simulink model "step2"  (R2018a)
settings: Solver=ode45  StartTime=0.0  StopTime=4  RelTol=1e-3
values from neighbouring files (symbols this model uses):
  Beta = 0    [step2.m]
  Friction = 22600    [step2.m]
  Inertia = 250000    [step2.m]
  Lambdam = 14.3522    [step2.m]
  Ld = 0.0035218    [step2.m]
  Lq = 0.0035218    [step2.m]
  Pole = 118    [step2.m]
  R = 58    [step2.m]
  Ro = 1.225    [step2.m]
  Rs = 0.05    [step2.m]
  Vw = 11.8    [step2.m]
libraries: powerlib x17, peTransforms x2
settings Model: Creator=Xinyi Zhang  LastModifiedBy=zxyxi

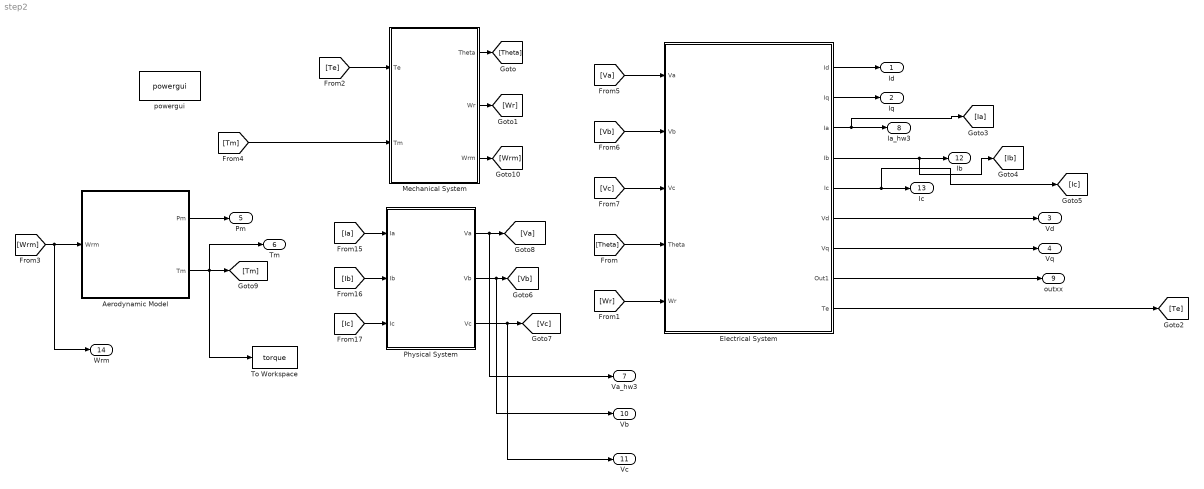
== system step2 ==
  "Aerodynamic Model " : Subsystem
  "Electrical System " : Subsystem
  "Mechanical System " : Subsystem
  "Physical System " : Subsystem
  To Workspace : ToWorkspace  VariableName=torque  SaveFormat=Timeseries  SampleTime=-1
  powergui : powerlib/powergui  Priority=1  SimulationMode=Discrete  SampleTime=50e-6  frequency=60  Iterations=50  frequencyindice=0  Pbase=100e6  ErrMax=1e-4  UnitsV=kV  UnitsW=MW  buscounter=0  FunctionMessages=off  echomessages=off  EnableUseOfTLC=off  CurrentSourceSwitches=off  DisableSnubberDevices=off  DisableRonSwitches=off  DisableVfSwitches=off  DisplayEquations=off  SolverType=Tustin/Backward Euler (TBE)  Interpol=off  ExternalGateDelay=off  methode=off  Ts=100  x0status=blocks  SPID=on  SwTol=0  HookPort=off  RestoreLinks=warning  ResistiveCurrentMeasurement=off  Frange=[0:2:500]  Ylog=off  Xlog=on  ShowGrid=off  save=off  variable=ZData  structure=0  ZoomFFT=off  StartTime=0.0  cycles=1  DisplayStyle=1  fundamental=60  FreqAxis=off  MaxFrequency=1000  frequencyindicesteady=1  RmsSteady=1  display=off
  Id : Outport
  Iq : Outport  Port=2
  "Vd " : Outport  Port=3
  "Vq " : Outport  Port=4
  Pm : Outport  Port=5
  Tm : Outport  Port=6
  "Va_hw3 " : Outport  Port=7
  "Ia_hw3 " : Outport  Port=8
  outxx : Outport  Port=9
  "Vb " : Outport  Port=10
  "Vc " : Outport  Port=11
  Ib : Outport  Port=12
  "Ic " : Outport  Port=13
  "Wrm " : Outport  Port=14
  wires:
  "Mechanical System "/1(Theta) -> [Theta]
  [Theta] -> "Electrical System "/4(Theta)
  [Wr] -> "Electrical System "/5(Wr)
  [Va] -> "Electrical System "/1(Va)
  [Vb] -> "Electrical System "/2(Vb)
  [Vc] -> "Electrical System "/3(Vc)
  "Mechanical System "/2(Wr) -> [Wr]
  "Electrical System "/1(Id) -> Id/1
  "Electrical System "/2(Iq) -> Iq/1
  [Ia] -> "Physical System "/1("Ia ")
  [Ib] -> "Physical System "/2("Ib ")
  [Ic] -> "Physical System "/3("Ic ")
  "Physical System "/1("Va ") -> "Va_hw3 "/1, [Va]
  "Physical System "/2("Vb ") -> "Vb "/1, [Vb]
  "Physical System "/3("Vc ") -> "Vc "/1, [Vc]
  [Te] -> "Mechanical System "/1(Te)
  "Electrical System "/4(Ib) -> Ib/1, [Ib]
  "Electrical System "/6("Vd ") -> "Vd "/1
  "Electrical System "/7("Vq ") -> "Vq "/1
  [Wrm] -> "Wrm "/1, "Aerodynamic Model "/1("Wrm ")
  "Aerodynamic Model "/1(Pm) -> Pm/1
  "Aerodynamic Model "/2(Tm) -> To Workspace/1, Tm/1, [Tm]
  "Mechanical System "/3("Wrm ") -> [Wrm]
  "Electrical System "/3(Ia) -> "Ia_hw3 "/1, [Ia]
  "Electrical System "/8(Out1) -> outxx/1
  "Electrical System "/9("Te ") -> [Te]
  [Tm] -> "Mechanical System "/2("Tm ")
  "Electrical System "/5(Ic) -> [Ic], "Ic "/1

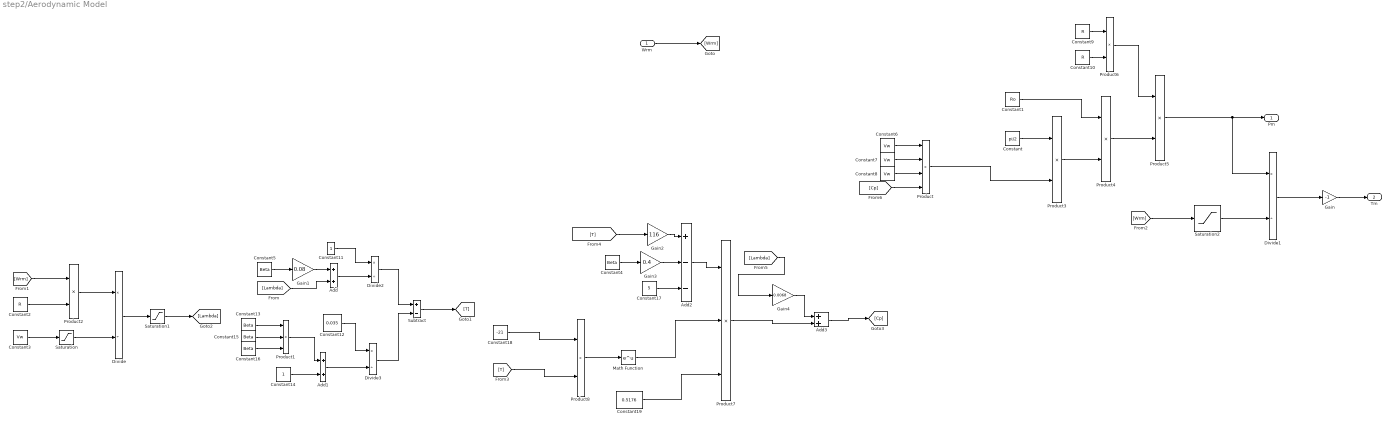
== system step2/Aerodynamic Model  ==
  "Wrm " : Inport
  Add : Sum
  Add1 : Sum
  Add2 : Sum  Inputs=+--
  Add3 : Sum
  Constant : Constant  Value=pi/2
  Constant1 : Constant  Value=Ro
  Constant10 : Constant  Value=R
  Constant11 : Constant
  Constant12 : Constant  Value=0.035
  Constant{4..5,13,15..16} (5 alike) : Constant  Value=Beta
  Constant14 : Constant
  Constant17 : Constant  Value=5
  Constant18 : Constant  Value=-21
  Constant19 : Constant  Value=0.5176
  Constant2 : Constant  Value=R
  Constant{3,6..8} (4 alike) : Constant  Value=Vw
  Constant9 : Constant  Value=R
  Divide{,1..3} (4 alike) : Product  Inputs=*/
  Gain : Gain  Gain=-1
  Gain1 : Gain  Gain=0.08
  Gain2 : Gain  Gain=116
  Gain3 : Gain  Gain=0.4
  Gain4 : Gain  Gain=0.0068
  Math Function : Math  SaturateOnIntegerOverflow=on
  Product : Product  Inputs=4
  Product1 : Product  Inputs=3
  Product{2..6,8} (6 alike) : Product
  Product7 : Product  Inputs=3
  Saturation : Saturate  UpperLimit=1e6  LowerLimit=1e-6
  Saturation1 : Saturate  UpperLimit=1e6  LowerLimit=1e-6
  Saturation2 : Saturate  UpperLimit=1e6  LowerLimit=1e-6
  Subtract : Sum  Inputs=+-
  Pm : Outport
  Tm : Outport  Port=2
  wires:
  [Wrm] -> Product2/1
  "Wrm "/1 -> [Wrm]
  Product2/1 -> Divide/1
  Saturation/1 -> Divide/2
  Divide/1 -> Saturation1/1
  Constant/1 -> Product3/1
  Product3/1 -> Product4/2
  Constant1/1 -> Product4/1
  Product4/1 -> Product5/2
  Product6/1 -> Product5/1
  Product5/1 -> Divide1/1, Pm/1
  Saturation2/1 -> Divide1/2
  Divide1/1 -> Gain/1
  Gain/1 -> Tm/1
  Constant2/1 -> Product2/2
  Constant3/1 -> Saturation/1
  Constant8/1 -> Product/3
  Constant7/1 -> Product/2
  Constant6/1 -> Product/1
  Constant9/1 -> Product6/1
  Constant10/1 -> Product6/2
  Product/1 -> Product3/2
  [Wrm] -> Saturation2/1
  Constant5/1 -> Gain1/1
  Gain1/1 -> Add/1
  [Lambda] -> Add/2
  Add/1 -> Divide2/2
  Constant11/1 -> Divide2/1
  Add1/1 -> Divide3/2
  Product1/1 -> Add1/1
  Constant12/1 -> Divide3/1
  Constant14/1 -> Add1/2
  Constant13/1 -> Product1/1
  Constant15/1 -> Product1/2
  Constant16/1 -> Product1/3
  Divide2/1 -> Subtract/1
  Divide3/1 -> Subtract/2
  Subtract/1 -> [T]
  Saturation1/1 -> [Lambda]
  Gain2/1 -> Add2/1
  [T] -> Gain2/1
  Constant4/1 -> Gain3/1
  Gain3/1 -> Add2/2
  Constant17/1 -> Add2/3
  Add2/1 -> Product7/1
  Math Function/1 -> Product7/2
  Constant19/1 -> Product7/3
  Product7/1 -> Add3/2
  [Lambda] -> Gain4/1
  Gain4/1 -> Add3/1
  Add3/1 -> [Cp]
  [Cp] -> Product/4
  Product8/1 -> Math Function/1
  Constant18/1 -> Product8/1
  [T] -> Product8/2

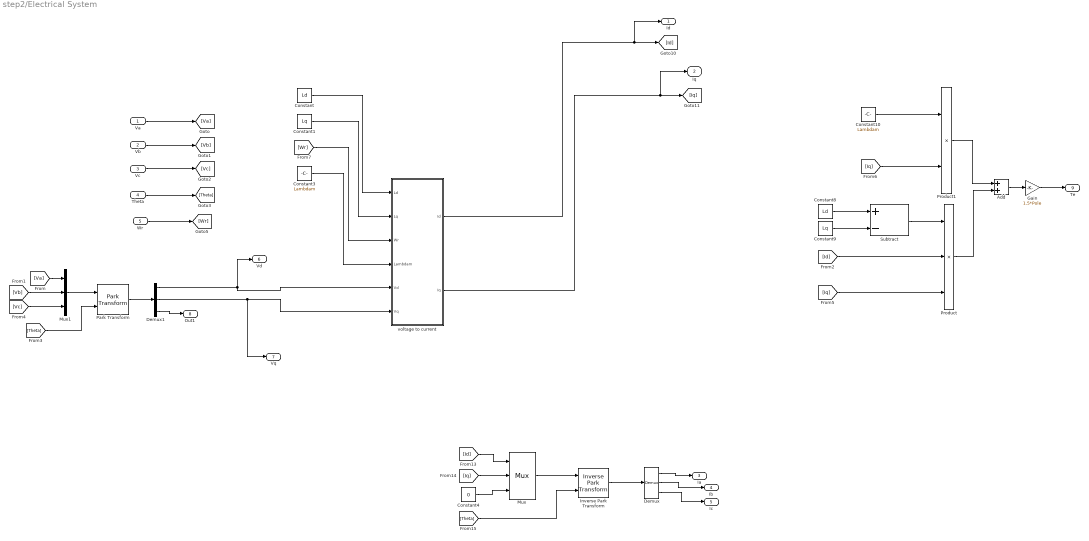
== system step2/Electrical System  ==
  Va : Inport
  Vb : Inport  Port=2
  Vc : Inport  Port=3
  Theta : Inport  Port=4
  Wr : Inport  Port=5
  Add : Sum
  Constant : Constant  Value=Ld
  Constant1 : Constant  Value=Lq
  Constant10 : Constant  Value=Lambdam
  Constant3 : Constant  Value=Lambdam
  Constant4 : Constant  Value=0
  Constant8 : Constant  Value=Ld
  Constant9 : Constant  Value=Lq
  Demux : Demux  Outputs=3
  Demux1 : Demux  Outputs=3
  Gain : Gain  Gain=1.5*Pole
  Inverse Park Transform : peTransforms/Inverse Park Transform  AxisAlignment=D-axis  PowerInvariant=off
  Mux : Mux  Inputs=3
  Mux1 : Mux  Inputs=3
  Park Transform : peTransforms/Park Transform  AxisAlignment=D-axis  PowerInvariant=off
  Product : Product  Inputs=3
  Product1 : Product
  Subtract : Sum  Inputs=+-
  voltage to current : Subsystem
  Id : Outport
  Iq : Outport  Port=2
  Ia : Outport  Port=3
  Ib : Outport  Port=4
  Ic : Outport  Port=5
  "Vd " : Outport  Port=6
  "Vq " : Outport  Port=7
  Out1 : Outport  Port=8
  "Te " : Outport  Port=9
  wires:
  Va/1 -> [Va]
  Vb/1 -> [Vb]
  Vc/1 -> [Vc]
  Theta/1 -> [Theta]
  Wr/1 -> [Wr]
  [Wr] -> voltage to current/3(Wr)
  Constant/1 -> voltage to current/1(Ld)
  Constant1/1 -> voltage to current/2("Lq ")
  Constant3/1 -> voltage to current/4(Lambdam)
  voltage to current/1(Id) -> Id/1, [Id]
  voltage to current/2(Iq) -> Iq/1, [Iq]
  [Id] -> Mux/1
  [Iq] -> Mux/2
  Constant4/1 -> Mux/3
  Demux/1 -> Ia/1
  Demux/2 -> Ib/1
  Demux/3 -> Ic/1
  [Va] -> Mux1/1
  [Vb] -> Mux1/2
  [Vc] -> Mux1/3
  Demux1/1 -> voltage to current/5("Vd "), "Vd "/1
  Demux1/2 -> "Vq "/1, voltage to current/6(Vq)
  Mux/1 -> Inverse Park Transform/1
  Inverse Park Transform/1 -> Demux/1
  [Theta] -> Inverse Park Transform/2
  Mux1/1 -> Park Transform/1
  [Theta] -> Park Transform/2
  Park Transform/1 -> Demux1/1
  Demux1/3 -> Out1/1
  Product/1 -> Add/2
  Add/1 -> Gain/1
  Product1/1 -> Add/1
  Constant9/1 -> Subtract/2
  Subtract/1 -> Product/1
  Gain/1 -> "Te "/1
  [Iq] -> Product/3
  Constant8/1 -> Subtract/1
  Constant10/1 -> Product1/1
  [Id] -> Product/2
  [Iq] -> Product1/2

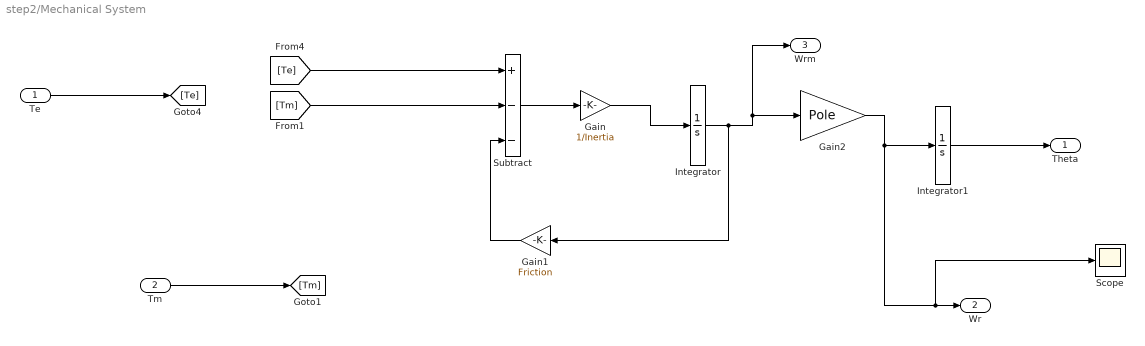
== system step2/Mechanical System  ==
  Te : Inport
  "Tm " : Inport  Port=2
  Gain : Gain  Gain=1/Inertia
  Gain1 : Gain  Gain=Friction
  Gain2 : Gain  Gain=Pole
  Integrator : Integrator
  Integrator1 : Integrator
  Scope : Scope
  Subtract : Sum  Inputs=+--
  Theta : Outport
  Wr : Outport  Port=2
  "Wrm " : Outport  Port=3
  wires:
  Integrator1/1 -> Theta/1
  Gain2/1 -> Scope/1, Wr/1, Integrator1/1
  Integrator/1 -> "Wrm "/1, Gain2/1, Gain1/1
  [Te] -> Subtract/1
  Te/1 -> [Te]
  Subtract/1 -> Gain/1
  Gain/1 -> Integrator/1
  Gain1/1 -> Subtract/3
  "Tm "/1 -> [Tm]
  [Tm] -> Subtract/2

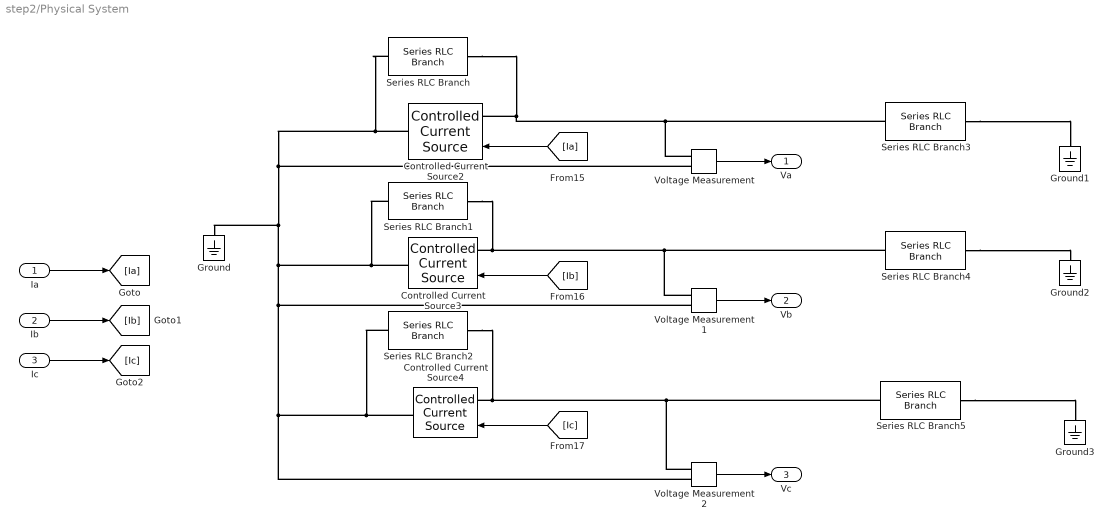
== system step2/Physical System  ==
  "Ia " : Inport
  "Ib " : Inport  Port=2
  "Ic " : Inport  Port=3
  Controlled Current Source2 : powerlib/Electrical Sources/Controlled Current Source  Initialize=on  Source_Type=AC  Amplitude=0  Phase=0  Frequency=0  Measurements=None
  Controlled Current Source3 : powerlib/Electrical Sources/Controlled Current Source  Initialize=on  Source_Type=AC  Amplitude=0  Phase=0  Frequency=0  Measurements=None
  Controlled Current Source4 : powerlib/Electrical Sources/Controlled Current Source  Initialize=on  Source_Type=AC  Amplitude=0  Phase=0  Frequency=0  Measurements=None
  Ground{,1..3} (4 alike) : powerlib/Elements/Ground  LConnTagsString=a
  Series RLC Branch : powerlib/Elements/Series RLC Branch  LConnTagsString=__new0  RConnTagsString=__new0  BranchType=R  Resistance=1000000  Inductance=1e-3  SetiL0=off  InitialCurrent=0  Capacitance=1e-6  Setx0=off  InitialVoltage=0  Measurements=None
  Series RLC Branch1 : powerlib/Elements/Series RLC Branch  LConnTagsString=__new0  RConnTagsString=__new0  BranchType=R  Resistance=1000000  Inductance=1e-3  SetiL0=off  InitialCurrent=0  Capacitance=1e-6  Setx0=off  InitialVoltage=0  Measurements=None
  Series RLC Branch2 : powerlib/Elements/Series RLC Branch  LConnTagsString=__new0  RConnTagsString=__new0  BranchType=R  Resistance=1000000  Inductance=1e-3  SetiL0=off  InitialCurrent=0  Capacitance=1e-6  Setx0=off  InitialVoltage=0  Measurements=None
  Series RLC Branch3 : powerlib/Elements/Series RLC Branch  LConnTagsString=__new0  RConnTagsString=__new0  BranchType=R  Resistance=10  Inductance=1e-3  SetiL0=off  InitialCurrent=0  Capacitance=1e-6  Setx0=off  InitialVoltage=0  Measurements=None
  Series RLC Branch4 : powerlib/Elements/Series RLC Branch  LConnTagsString=__new0  RConnTagsString=__new0  BranchType=R  Resistance=10  Inductance=1e-3  SetiL0=off  InitialCurrent=0  Capacitance=1e-6  Setx0=off  InitialVoltage=0  Measurements=None
  Series RLC Branch5 : powerlib/Elements/Series RLC Branch  LConnTagsString=__new0  RConnTagsString=__new0  BranchType=R  Resistance=10  Inductance=1e-3  SetiL0=off  InitialCurrent=0  Capacitance=1e-6  Setx0=off  InitialVoltage=0  Measurements=None
  Voltage Measurement : powerlib/Measurements/Voltage Measurement  PhasorSimulation=off  OutputType=Complex  PSBequivalent=0
  Voltage Measurement1 : powerlib/Measurements/Voltage Measurement  PhasorSimulation=off  OutputType=Complex  PSBequivalent=0
  Voltage Measurement2 : powerlib/Measurements/Voltage Measurement  PhasorSimulation=off  OutputType=Complex  PSBequivalent=0
  "Va " : Outport
  "Vb " : Outport  Port=2
  "Vc " : Outport  Port=3
  wires:
  [Ib] -> Controlled Current Source3/1
  [Ia] -> Controlled Current Source2/1
  [Ic] -> Controlled Current Source4/1
  "Ia "/1 -> [Ia]
  "Ib "/1 -> [Ib]
  "Ic "/1 -> [Ic]
  Voltage Measurement/1 -> "Va "/1
  Voltage Measurement1/1 -> "Vb "/1
  Voltage Measurement2/1 -> "Vc "/1
  connections:
  Controlled Current Source2/RConn1 -- Series RLC Branch/LConn1 -- Voltage Measurement2/LConn2 -- Series RLC Branch2/LConn1 -- Controlled Current Source4/RConn1 -- Voltage Measurement1/LConn2 -- Series RLC Branch1/LConn1 -- Controlled Current Source3/RConn1 -- Ground/LConn1 -- Voltage Measurement/LConn2
  Series RLC Branch/RConn1 -- Voltage Measurement/LConn1 -- Series RLC Branch3/LConn1 -- Controlled Current Source2/LConn1
  Series RLC Branch1/RConn1 -- Voltage Measurement1/LConn1 -- Series RLC Branch4/LConn1 -- Controlled Current Source3/LConn1
  Series RLC Branch2/RConn1 -- Voltage Measurement2/LConn1 -- Series RLC Branch5/LConn1 -- Controlled Current Source4/LConn1
  Series RLC Branch3/RConn1 -- Ground1/LConn1
  Series RLC Branch4/RConn1 -- Ground2/LConn1
  Series RLC Branch5/RConn1 -- Ground3/LConn1

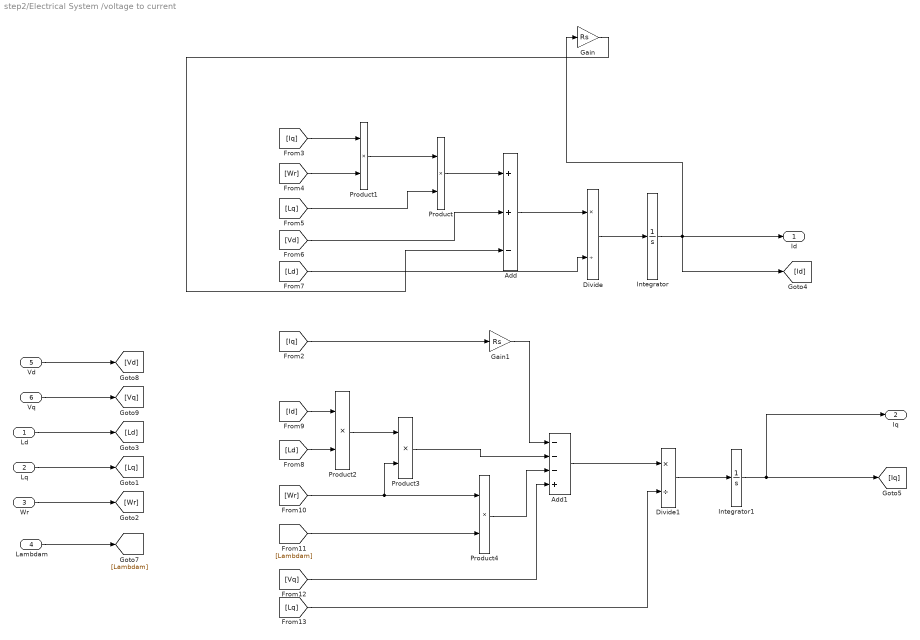
== system step2/Electrical System /voltage to current ==
  Ld : Inport
  "Lq " : Inport  Port=2
  Wr : Inport  Port=3
  Lambdam : Inport  Port=4
  "Vd " : Inport  Port=5
  Vq : Inport  Port=6
  Add : Sum  Inputs=++-
  Add1 : Sum  Inputs=---+
  Divide : Product  Inputs=*/
  Divide1 : Product  Inputs=*/
  Gain : Gain  Gain=Rs
  Gain1 : Gain  Gain=Rs
  Integrator : Integrator
  Integrator1 : Integrator
  Product{,1..4} (5 alike) : Product
  Id : Outport
  Iq : Outport  Port=2
  wires:
  Integrator/1 -> [Id], Gain/1, Id/1
  [Wr] -> Product3/2, Product4/1
  Product2/1 -> Product3/1
  Product1/1 -> Product/1
  Divide1/1 -> Integrator1/1
  Add/1 -> Divide/1
  [Id] -> Product2/1
  [Lambdam] -> Product4/2
  Divide/1 -> Integrator/1
  Integrator1/1 -> Iq/1, [Iq]
  [Iq] -> Product1/1
  [Wr] -> Product1/2
  [Lq] -> Product/2
  [Ld] -> Divide/2
  Product3/1 -> Add1/2
  [Vd] -> Add/2
  Add1/1 -> Divide1/1
  [Lq] -> Divide1/2
  [Ld] -> Product2/2
  Product/1 -> Add/1
  Product4/1 -> Add1/3
  [Vq] -> Add1/4
  Wr/1 -> [Wr]
  Ld/1 -> [Ld]
  "Lq "/1 -> [Lq]
  Lambdam/1 -> [Lambdam]
  "Vd "/1 -> [Vd]
  Vq/1 -> [Vq]
  Gain/1 -> Add/3
  [Iq] -> Gain1/1
  Gain1/1 -> Add1/1
